simulink model "Damper_usingcurrent"  (Simulink 10.2)
settings: Solver=ode4  StartTime=0.0  StopTime=10.0  FixedStep=0.0001  RelTol=1e-3
libraries: simulink x2
settings Model: Creator=lenovo  LastModifiedBy=lenovo
settings DataIOCC: SaveFormat=Dataset  SignalLoggingSaveFormat=Dataset  ReturnWorkspaceOutputs=on
settings OptimizationCC: LifeSpan=auto
settings DebuggingCC: UnderspecifiedInitializationDetection=Simplified  MergeDetectMultiDrivingBlocksExec=error  FcnCallInpInsideContextMsg=error  SFUnexpectedBacktrackingDiag=error  SFNoUnconditionalDefaultTransitionDiag=error  SFExecutionAtInitializationDiag=warning  ArithmeticOperatorsInVariantConditions=error
settings HardwareCC: ProdBitPerPointer=64  ProdBitPerSizeT=64  ProdBitPerPtrDiffT=64  ProdLargestAtomicFloat=Float  ProdIntDivRoundTo=Zero  ProdEndianess=LittleEndian  ProdWordSize=64  ProdHWDeviceType=Intel->x86-64 (Windows64)
settings ModelReferenceCC: PropagateSignalLabelsOutOfModel=on
settings SFSimCC: SimUseLocalCustomCode=on  CustomCodeUndefinedFunction=FilterOut
settings RTWCC: RTWUseLocalCustomCode=on
settings CodeAppCC: StateflowObjectComments=off
settings GRTTargetCC: TargetLangStandard=C99 (ISO)  CombineOutputUpdateFcns=on  GRTInterface=off
settings ConfigComp: CovMetricSettings=dwe  CovSaveCumulativeToWorkspaceVar=off  CovSaveSingleToWorkspaceVar=off  CovExternalEMLEnable=on

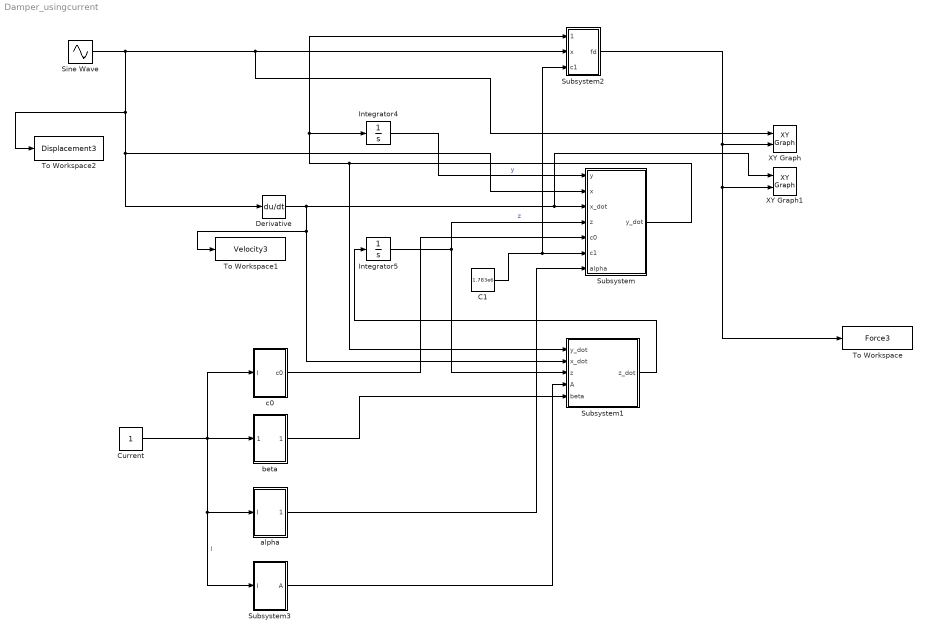
== system Damper_usingcurrent ==
  C1 : Constant  Value=1.783e6
  Current : Constant
  Derivative : Derivative
  Integrator4 : Integrator
  Integrator5 : Integrator
  Sine Wave : Sin  Amplitude=0.005  Frequency=pi  Phase=pi/2  SampleTime=0
  Subsystem : Subsystem
  Subsystem1 : Subsystem
  Subsystem2 : Subsystem
  Subsystem3 : Subsystem
  To Workspace : ToWorkspace  VariableName=Force3  SampleTime=-1
  To Workspace1 : ToWorkspace  VariableName=Velocity3  SampleTime=-1
  To Workspace2 : ToWorkspace  VariableName=Displacement3  SampleTime=-1
  XY Graph : simulink/Sinks/XY Graph  xmin=-0.005  xmax=0.005  ymin=-1  ymax=1  st=-1
  XY Graph1 : simulink/Sinks/XY Graph  xmin=-1  xmax=1  ymin=-1  ymax=1  st=-1
  alpha : Subsystem
  beta : Subsystem
  c0 : Subsystem
  wires:
  Subsystem3/1(A) -> Subsystem1/4(A)
  beta/1(Out1) -> Subsystem1/5(beta)
  alpha/1(Out1) -> Subsystem/7(alpha)
  Integrator4/1 -> Subsystem/1(y)  "y"
  Current/1 -> c0/1(I), beta/1(In1), Subsystem3/1(I), alpha/1(I)  "I"
  Sine Wave/1 -> To Workspace2/1, Derivative/1, Subsystem/2(x), XY Graph/1, Subsystem2/2(x)
  Subsystem2/1(fd) -> To Workspace/1, XY Graph1/2, XY Graph/2
  C1/1 -> Subsystem2/3(c1), Subsystem/6(c1)
  Integrator5/1 -> Subsystem1/3(z), Subsystem/4(z)  "z"
  Subsystem1/1(z_dot) -> Integrator5/1
  c0/1(c0) -> Subsystem/5(c0)
  Derivative/1 -> To Workspace1/1, Subsystem1/2(x_dot), XY Graph1/1, Subsystem/3(x_dot)
  Subsystem/1(y_dot) -> Subsystem1/1(y_dot), Integrator4/1, Subsystem2/1(y_dot)

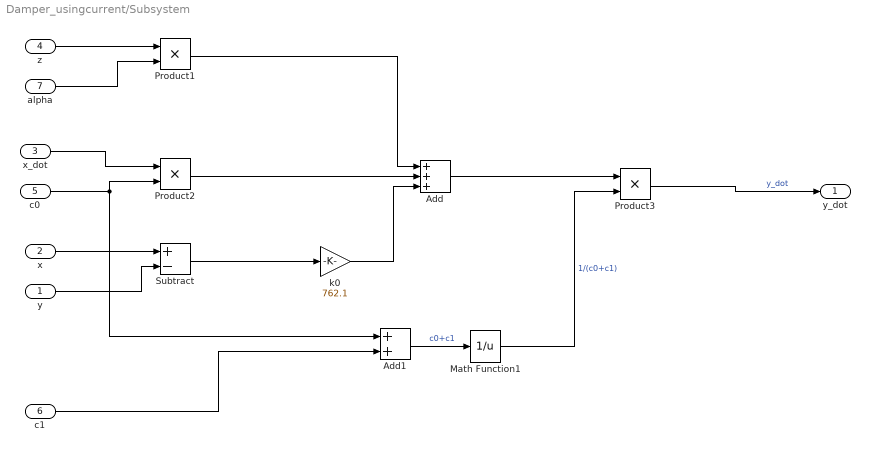
== system Damper_usingcurrent/Subsystem ==
  y : Inport
  x : Inport  Port=2
  x_dot : Inport  Port=3
  z : Inport  Port=4
  c0 : Inport  Port=5
  c1 : Inport  Port=6
  alpha : Inport  Port=7
  Add : Sum  Inputs=+++
  Add1 : Sum
  Math Function1 : Math  Operator=reciprocal  SaturateOnIntegerOverflow=on
  Product1 : Product
  Product2 : Product
  Product3 : Product
  Subtract : Sum  Inputs=+-
  k0 : Gain  Gain=762.1
  y_dot : Outport
  wires:
  Product1/1 -> Add/1
  Subtract/1 -> k0/1
  Add1/1 -> Math Function1/1  "c0+c1"
  k0/1 -> Add/3
  Math Function1/1 -> Product3/2  "1/(c0+c1)"
  c0/1 -> Add1/1, Product2/2
  z/1 -> Product1/1
  Product3/1 -> y_dot/1  "y_dot"
  Add/1 -> Product3/1
  Product2/1 -> Add/2
  y/1 -> Subtract/2
  x/1 -> Subtract/1
  c1/1 -> Add1/2
  x_dot/1 -> Product2/1
  alpha/1 -> Product1/2

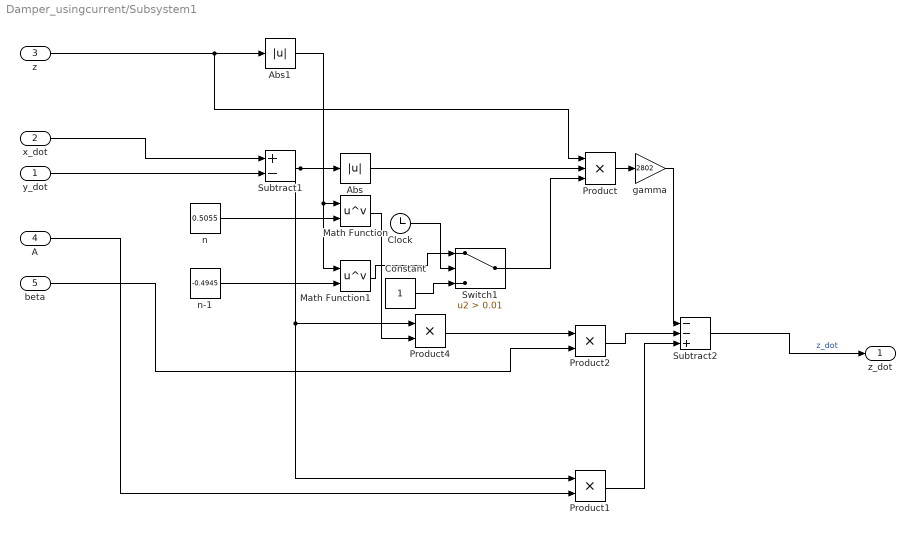
== system Damper_usingcurrent/Subsystem1 ==
  y_dot : Inport
  x_dot : Inport  Port=2
  z : Inport  Port=3
  A : Inport  Port=4
  beta : Inport  Port=5
  Abs : Abs
  Abs1 : Abs
  Clock : Clock
  Constant : Constant
  Math Function : Math  Operator=pow  SaturateOnIntegerOverflow=on
  Math Function1 : Math  Operator=pow  SaturateOnIntegerOverflow=on
  Product : Product  Inputs=3
  Product1 : Product
  Product2 : Product
  Product4 : Product
  Subtract1 : Sum  Inputs=+-
  Subtract2 : Sum  Inputs=--+
  Switch1 : Switch  Criteria=u2 > Threshold  Threshold=0.01
  gamma : Gain  Gain=2802
  n : Constant  Value=0.5055
  n-1 : Constant  Value=-0.4945
  z_dot : Outport
  wires:
  Abs/1 -> Product/2
  Subtract1/1 -> Product1/1, Product4/1, Abs/1
  n/1 -> Math Function/2
  Abs1/1 -> Math Function1/1, Math Function/1
  gamma/1 -> Subtract2/1
  z/1 -> Abs1/1, Product/1
  Product2/1 -> Subtract2/2
  Product4/1 -> Product2/1
  Math Function/1 -> Product4/2
  Product/1 -> gamma/1
  y_dot/1 -> Subtract1/2
  Subtract2/1 -> z_dot/1  "z_dot"
  x_dot/1 -> Subtract1/1
  Product1/1 -> Subtract2/3
  n-1/1 -> Math Function1/2
  A/1 -> Product1/2
  beta/1 -> Product2/2
  Math Function1/1 -> Switch1/1
  Switch1/1 -> Product/3
  Constant/1 -> Switch1/3
  Clock/1 -> Switch1/2

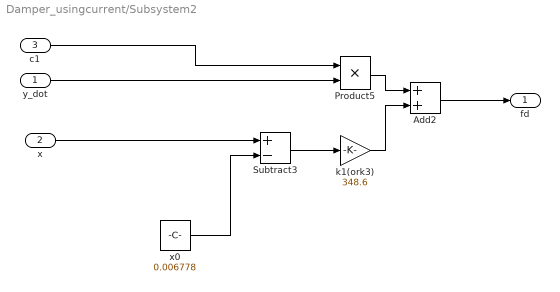
== system Damper_usingcurrent/Subsystem2 ==
  y_dot : Inport
  x : Inport  Port=2
  c1 : Inport  Port=3
  Add2 : Sum
  Product5 : Product
  Subtract3 : Sum  Inputs=+-
  k1(ork3) : Gain  Gain=348.6
  x0 : Constant  Value=0.006778
  fd : Outport
  wires:
  Subtract3/1 -> k1(ork3)/1
  y_dot/1 -> Product5/2
  Product5/1 -> Add2/1
  k1(ork3)/1 -> Add2/2
  Add2/1 -> fd/1
  x0/1 -> Subtract3/2
  c1/1 -> Product5/1
  x/1 -> Subtract3/1

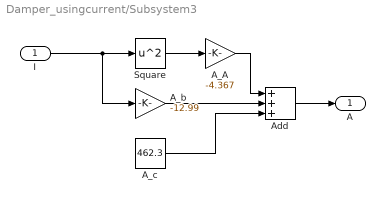
== system Damper_usingcurrent/Subsystem3 ==
  I : Inport
  A_A : Gain  Gain=-4.367
  A_b : Gain  Gain=-12.99
  A_c : Constant  Value=462.3
  Add : Sum  Inputs=+++
  Square : Math  Operator=square  SaturateOnIntegerOverflow=on
  A : Outport
  wires:
  I/1 -> A_b/1, Square/1
  Square/1 -> A_A/1
  A_b/1 -> Add/2
  A_A/1 -> Add/1
  Add/1 -> A/1
  A_c/1 -> Add/3

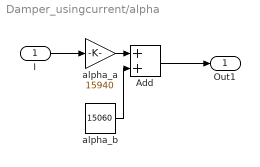
== system Damper_usingcurrent/alpha ==
  I : Inport
  Add : Sum
  alpha_a : Gain  Gain=15940
  alpha_b : Constant  Value=15060
  Out1 : Outport
  wires:
  I/1 -> alpha_a/1
  alpha_a/1 -> Add/1
  alpha_b/1 -> Add/2
  Add/1 -> Out1/1

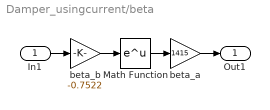
== system Damper_usingcurrent/beta ==
  In1 : Inport
  Math Function : Math  SaturateOnIntegerOverflow=on
  beta_a : Gain  Gain=1415
  beta_b : Gain  Gain=-0.7522
  Out1 : Outport
  wires:
  In1/1 -> beta_b/1
  beta_b/1 -> Math Function/1
  Math Function/1 -> beta_a/1
  beta_a/1 -> Out1/1

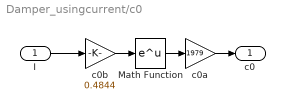
== system Damper_usingcurrent/c0 ==
  I : Inport
  Math Function : Math  SaturateOnIntegerOverflow=on
  c0a : Gain  Gain=1979
  c0b : Gain  Gain=0.4844
  c0 : Outport
  wires:
  c0b/1 -> Math Function/1
  I/1 -> c0b/1
  c0a/1 -> c0/1
  Math Function/1 -> c0a/1
